simulink model "sf_dcmotor"  (Simulink 7.6)
settings: Solver=ode45  StartTime=0.0  StopTime=10  RelTol=1e-3
settings Model: Creator=The MathWorks Inc.
settings OptimizationCC: InitFltsAndDblsToZero=on
settings DebuggingCC: SolverPrmCheckMsg=none  StrictBusMsg=Warning
settings SFSimCC: SimParseCustomCode=off

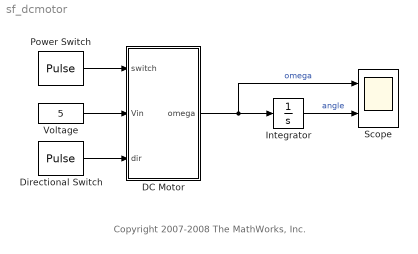
== system sf_dcmotor ==
  note: Copyright 2007-2008 The MathWorks, Inc.
  DC Motor : Subsystem  mask{R=2.0, L=0.5, Km=.015, Kb=.015, Kf=0.2, J=0.02}
      mask prompts: R "Resistance (Ohms)"; L "Inductance (Henrys)"; Km "Torque Constant"; Kb "EMF Constant"; Kf "Damping Constant"; J "Inertia"
  Directional Switch : DiscretePulseGenerator  PulseType=Time based  Period=1  PulseWidth=50
  Integrator : Integrator
  Power Switch : DiscretePulseGenerator  PulseType=Time based  Period=5  PulseWidth=50  PhaseDelay=2.5
  Scope : Scope  NumInputPorts=2
      settings: YMin=0.178025~-5  YMax=0.196765~5
  Voltage : Constant  Value=5
  wires:
  Voltage/1 -> DC Motor/2(Vin)
  DC Motor/1(omega) -> Integrator/1, Scope/1  "omega"
  Integrator/1 -> Scope/2  "angle"
  Directional Switch/1 -> DC Motor/3(dir)
  Power Switch/1 -> DC Motor/1(switch)

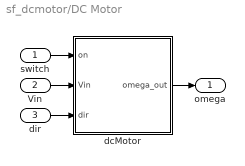
== system sf_dcmotor/DC Motor ==
  switch : Inport
  Vin : Inport  Port=2
  dir : Inport  Port=3
  dcMotor : Stateflow chart  TreatAsAtomicUnit=on
  omega : Outport
  wires:
  switch/1 -> dcMotor/1(on)
  dcMotor/1(omega_out) -> omega/1
  Vin/1 -> dcMotor/2(Vin)
  dir/1 -> dcMotor/3(dir)

== stateflow chart DC Motor/dcMotor ==
  settings: updateMethod=CONTINUOUS  initializeOutput=1
  state powerOn
    state down
      du:
      % Derivatives
      curr_dot = idotCalc(-Vin,curr,omega);
      omega_dot = wdotCalc(curr,omega);
      % Output
      omega_out=omega;
    state up
      du:
      % Derivatives
      curr_dot = idotCalc(Vin,curr,omega);
      omega_dot = wdotCalc(curr,omega);
      % Output
      omega_out=omega;
    down -> up : [dir==1]
    up -> down : [dir==0]
    (default) -> down [order 2]
    (default) -> up [order 1] : [dir == 1]
  state powerOff
    du:
    % Derivatives
    curr_dot = idotCalc(0,curr,omega);
    omega_dot = wdotCalc(curr,omega);
    % Output
    omega_out=omega;
  state der = idotCalc(volts,i,w) [function]
    (default) -> (junction 9) : {der=-R/L*i - Kb/L*w + 1.0/L*volts;}
  state der = wdotCalc(i,w) [function]
    (default) -> (junction 10) : {der=Km/J*i - Kf/J*w;}
  (default) -> powerOff : {curr=0;
      | omega=0;}
  powerOn -> powerOff : [!on]
  powerOff -> powerOn : [on]
  data: volts function_input double; der function_output double; i function_input double; w function_input double; der function_output double; i function_input double; w function_input double; curr local double; on input double; omega local double; omega_out output double; Vin input double; J parameter double =.02; Kb parameter double =.015; Kf parameter double =.2; Km parameter double =.015; L parameter double; R parameter double; dir input double
  data curr settings: updateMethod=SF_CONTINUOUS_TIME_DATA
  data omega settings: updateMethod=SF_CONTINUOUS_TIME_DATA
